simulink model "OMNIDUINO_4"  (R2017b)
settings: Solver=ode45  StartTime=0.0  StopTime=10  MaxStep=0.001  RelTol=1e-3  EnableMultiTasking=on
InitFcn:
  | Simu_Omniduino_4;
values from neighbouring files (symbols this model uses):
  centerX = 0    [Simu_Omniduino_4.m]
  centerY = 0    [Simu_Omniduino_4.m]
  DER_GAIN = 2    [Simu_Omniduino_4.m]
  LOW_SAT_LIM = [-0.0625 -0.0625 -10]    [Simu_Omniduino_4.m]
  phaseX = pi/2    (= 1.57079632679)    [Simu_Omniduino_4.m]
  phaseY = 0    [Simu_Omniduino_4.m]
  PROP_GAIN = [1.5 1.5 1.5]    [Simu_Omniduino_4.m]
  R = 0.5    [Simu_Omniduino_4.m]
  T = 80/(2*pi*WR) * [0, -1, -D; 0.5.*sqrt(3), 0.5, -D; -0.5*sqrt(3), 0.5, -D]    [Simu_Omniduino_4.m]
  Tr = 0.015    [Simu_Omniduino_4.m]
  Ts = 0.125    [Simu_Omniduino_4.m]
  UPPR_SAT_LIM = [0.0625 0.0625 10]    [Simu_Omniduino_4.m]
  V = 0.35    [Simu_Omniduino_4.m]
undefined symbols (not defined in the file or in its folder): DiscIntNeverNeededParam
libraries: simulink x3, robotcorelib x2, peGeneralControl x1
settings Model: Creator=Fran  LastModifiedBy=fran
settings SolverCC: ZeroCrossControl=DisableAll
settings DataIOCC: LimitDataPoints=on  SaveFormat=Array
settings OptimizationCC: LifeSpan=inf
settings DebuggingCC: SFUnexpectedBacktrackingDiag=warning  SFNoUnconditionalDefaultTransitionDiag=warning  SFExecutionAtInitializationDiag=none
settings HardwareCC: ProdBitPerPointer=32  ProdBitPerSizeT=32  ProdBitPerPtrDiffT=32  ProdLargestAtomicFloat=None  ProdIntDivRoundTo=Undefined  ProdEndianess=Unspecified  ProdWordSize=32  ProdHWDeviceType=32-bit Generic
settings ModelReferenceCC: PropagateSignalLabelsOutOfModel=off
settings CodeAppCC: StateflowObjectComments=on
settings GRTTargetCC: TargetLangStandard=C89/C90 (ANSI)  GeneratePreprocessorConditionals=Disable all
settings ConfigComp: CovMetricSettings=dw  CovHtmlReporting=on  CovSaveCumulativeToWorkspaceVar=on  CovSaveSingleToWorkspaceVar=on  CovExternalEMLEnable=off

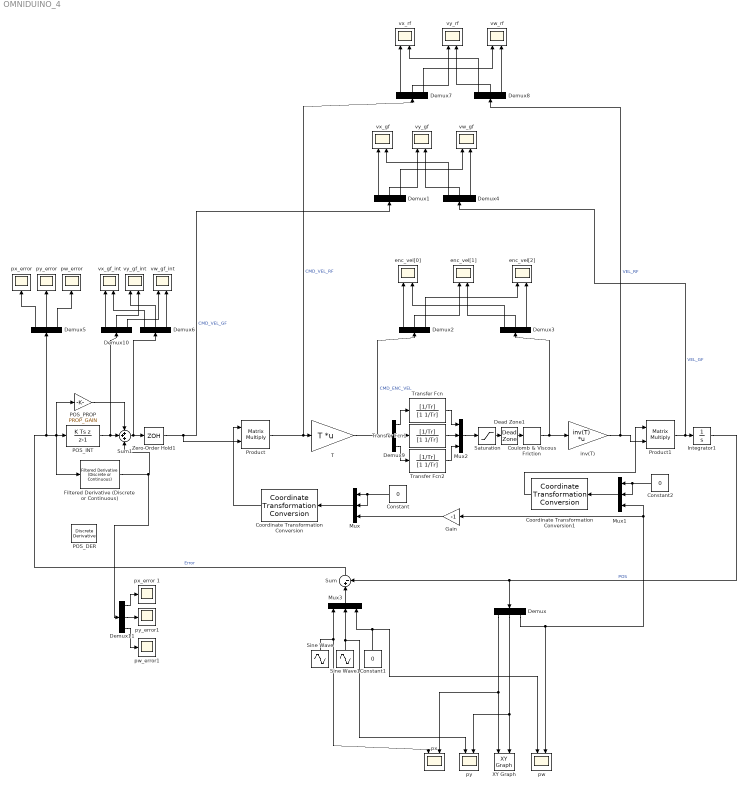
== system OMNIDUINO_4 ==
  Constant : Constant  Value=0
  Constant1 : Constant  Value=0
  Constant2 : Constant  Value=0
  Coordinate Transformation Conversion : robotcorelib/Coordinate Transformation Conversion  InputRepresentation=Euler Angles  InputEulerSequence=XYZ  ShowTrVecInputPort=on  OutputRepresentation=Rotation Matrix  OutputEulerSequence=XYZ  ShowTrVecOutputPort=on  SimulateUsing=Interpreted execution
      settings: SourceProductBaseCode=RO
  Coordinate Transformation Conversion1 : robotcorelib/Coordinate Transformation Conversion  InputRepresentation=Euler Angles  InputEulerSequence=XYZ  ShowTrVecInputPort=on  OutputRepresentation=Rotation Matrix  OutputEulerSequence=XYZ  ShowTrVecOutputPort=on  SimulateUsing=Interpreted execution
      settings: SourceProductBaseCode=RO
  Coulomb & Viscous Friction : simulink/Discontinuities/Coulomb & Viscous Friction  offset=[10]  gain=1
      settings: SourceProductName=Simulink
  Dead Zone1 : DeadZone  LowerValue=-10  UpperValue=10  LinearizeAsGain=off  ZeroCross=off
  Demux{,1..11} (12 alike) : Demux  Outputs=3
  Filtered Derivative (Discrete or Continuous) : peGeneralControl/Filtered Derivative (Discrete or Continuous)  K=DER_GAIN  T=0.2  B=inf  A=-inf  minRatio=10  Ts=-1
  Gain : Gain  Gain=-1
  Integrator1 : Integrator  InitialCondition=[0.5; 0; 0]
  Mux{,1..3} (4 alike) : Mux  Inputs=3
  POS_DER : simulink/Discrete/Discrete Derivative  gainval=DER_GAIN  ICPrevScaledInput=0.0  InputProcessing=Inherited  OutMin=[]  OutMax=[]  OutDataType=fixdt(1, 16)  OutScaling=2^-10  DoSatur=off
  POS_INT : DiscreteIntegrator  IntegratorMethod=Integration: Backward Euler  gainval=INT_GAIN  InitialConditionSetting=State (most efficient)  SampleTime=-1  SaturateOnIntegerOverflow=on  LimitOutput=on  UpperSaturationLimit=UPPR_SAT_LIM  LowerSaturationLimit=LOW_SAT_LIM  ICPrevOutput=DiscIntNeverNeededParam  ICPrevScaledInput=DiscIntNeverNeededParam
  POS_PROP : Gain  Gain=PROP_GAIN
  Product : Product  Multiplication=Matrix(*)
  Product1 : Product  Multiplication=Matrix(*)
  Saturation : Saturate  UpperLimit=160  LowerLimit=-160  ZeroCross=off
  Sine Wave : Sin  Amplitude=R  Bias=centerX  Frequency=V/R  Phase=phaseX  SampleTime=0
  Sine Wave1 : Sin  Amplitude=R  Bias=centerY  Frequency=V/R  Phase=phaseY  SampleTime=0
  Sum : Sum  Inputs=|+-
  Sum1 : Sum  Inputs=+++
  T : Gain  Gain=T  Multiplication=Matrix(K*u) (u vector)
  Transfer Fcn : TransferFcn  Numerator=[1/Tr]  Denominator=[1 1/Tr]
  Transfer Fcn1 : TransferFcn  Numerator=[1/Tr]  Denominator=[1 1/Tr]
  Transfer Fcn2 : TransferFcn  Numerator=[1/Tr]  Denominator=[1 1/Tr]
  XY Graph : simulink/Sinks/XY Graph  xmin=-1.5  xmax=1.5  ymin=-1.5  ymax=1.5  st=-1
  Zero-Order Hold1 : ZeroOrderHold  SampleTime=Ts
  enc_vel[0] : Scope  NumInputPorts=2
  enc_vel[1] : Scope  NumInputPorts=2
  enc_vel[2] : Scope  NumInputPorts=2
  inv(T) : Gain  Gain=inv(T)  Multiplication=Matrix(K*u) (u vector)
  pw : Scope  NumInputPorts=2
  pw_error : Scope
  pw_error1 : Scope
  px : Scope  NumInputPorts=2
  "px_error " : Scope
  px_error 1 : Scope
  py : Scope  NumInputPorts=2
  py_error : Scope
  py_error1 : Scope
  vw_gf : Scope  NumInputPorts=2
  vw_gf_int : Scope  NumInputPorts=2
  vw_rf : Scope  NumInputPorts=2
  vx_gf : Scope  NumInputPorts=2
  "vx_gf_int " : Scope  NumInputPorts=2
  vx_rf : Scope  NumInputPorts=2
  vy_gf : Scope  NumInputPorts=2
  vy_gf_int : Scope  NumInputPorts=2
  "vy_rf " : Scope  NumInputPorts=2
  wires:
  Integrator1/1 -> Sum/2, Demux/1  "POS"
  Sum/1 -> Demux5/1, Filtered Derivative (Discrete or Continuous)/1, POS_INT/1, POS_PROP/1  "Error"
  Demux/2 -> py/2, XY Graph/2
  Demux/1 -> px/2, XY Graph/1
  Demux1/2 -> vy_gf/1
  Demux1/1 -> vx_gf/1
  Demux2/1 -> enc_vel[0]/1
  T/1 -> Demux9/1, Demux2/1  "CMD_ENC_VEL"
  Demux2/2 -> enc_vel[1]/1
  Demux2/3 -> enc_vel[2]/1
  Demux3/1 -> enc_vel[0]/2
  Demux3/2 -> enc_vel[1]/2
  Demux3/3 -> enc_vel[2]/2
  Sum1/1 -> Zero-Order Hold1/1, Demux6/1
  POS_PROP/1 -> Sum1/1
  POS_INT/1 -> Demux10/1, Sum1/2
  Demux4/1 -> vx_gf/2
  Demux4/2 -> vy_gf/2
  Demux5/1 -> "px_error "/1
  Demux5/2 -> py_error/1
  Demux6/2 -> vy_gf_int/1
  Demux6/3 -> vw_gf_int/2
  Demux1/3 -> vw_gf/1
  Demux4/3 -> vw_gf/2
  Mux/1 -> Coordinate Transformation Conversion/1
  Product/1 -> Demux7/1, T/1  "CMD_VEL_RF"
  Coordinate Transformation Conversion/1 -> Product/1
  Zero-Order Hold1/1 -> Demux1/1, Product/2  "CMD_VEL_GF"
  Constant2/1 -> Mux1/2, Mux1/1
  Mux1/1 -> Coordinate Transformation Conversion1/1
  Product1/1 -> Demux4/1, Integrator1/1  "VEL_GF"
  Coordinate Transformation Conversion1/1 -> Product1/1
  inv(T)/1 -> Product1/2, Demux8/1  "VEL_RF"
  Demux7/1 -> vx_rf/1
  Demux7/3 -> vw_rf/1
  Demux7/2 -> "vy_rf "/1
  Demux8/2 -> "vy_rf "/2
  Demux8/1 -> vx_rf/2
  Constant/1 -> Mux/2, Mux/1
  Demux/3 -> pw/2, Mux1/3, Gain/1
  Demux5/3 -> pw_error/1
  Gain/1 -> Mux/3
  Demux9/2 -> Transfer Fcn1/1
  Demux9/1 -> Transfer Fcn/1
  Transfer Fcn/1 -> Mux2/1
  Transfer Fcn1/1 -> Mux2/2
  Transfer Fcn2/1 -> Mux2/3
  Demux9/3 -> Transfer Fcn2/1
  Coulomb & Viscous Friction/1 -> inv(T)/1, Demux3/1
  Mux2/1 -> Saturation/1
  Saturation/1 -> Dead Zone1/1
  Dead Zone1/1 -> Coulomb & Viscous Friction/1
  Mux3/1 -> Sum/1
  Sine Wave/1 -> Mux3/1, px/1
  Constant1/1 -> pw/1, Mux3/3
  Sine Wave1/1 -> Mux3/2, py/1
  Demux8/3 -> vw_rf/2
  Demux6/1 -> "vx_gf_int "/2
  Demux10/3 -> vw_gf_int/1
  Demux10/2 -> vy_gf_int/2
  Demux10/1 -> "vx_gf_int "/1
  Demux11/1 -> px_error 1/1
  Demux11/2 -> py_error1/1
  Demux11/3 -> pw_error1/1
  Filtered Derivative (Discrete or Continuous)/1 -> Demux11/1, Sum1/3
